simulink model "Close_Loop"  (R2019a)
settings: Solver=FixedStepDiscrete  StartTime=0.0  StopTime=100  RelTol=1e-3
libraries: simulink x5, slctrlblks x2
settings Model: Creator=markd  LastModifiedBy=lenovo
settings DebuggingCC: UnderSpecifiedDimensionMsg=warning

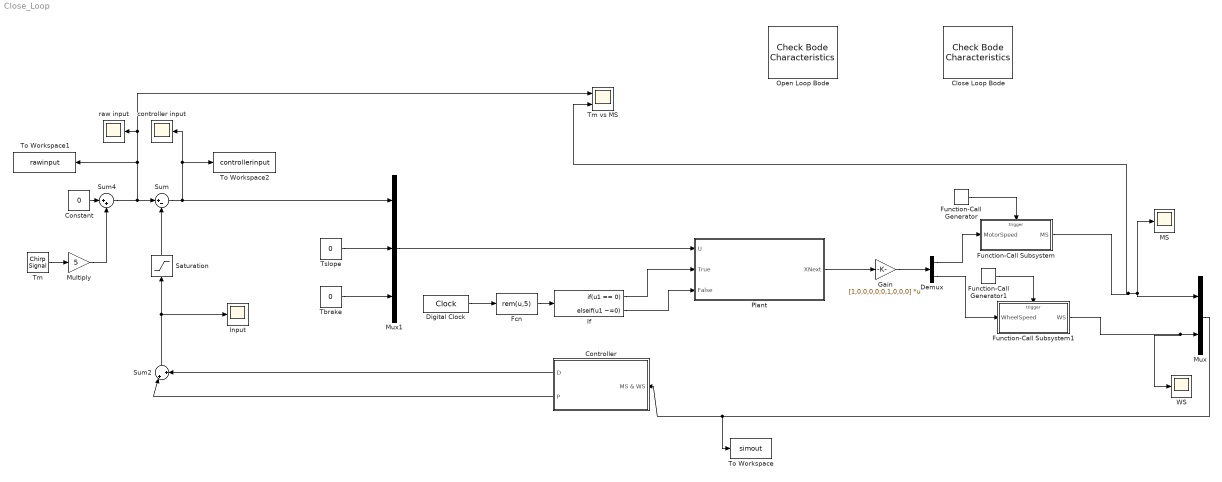
== system Close_Loop ==
  Close Loop Bode : slctrlblks/Model Verification/Check Bode  Characteristics  InstantiateOnLoad=on  SaveOperatingPoints=off  LinearizationIOs={'/Sum', 1, 'in', 'off', '';'/Demux', 1, 'out', 'off', ''}  LinearizeAt=SnapshotTimes  SnapshotTimes=[0]  TriggerType=rising  SampleTime=auto  RateConversionMethod=zoh  PreWarpFreq=10  UseExactDelayModel=off  UseFullBlockNameLabels=off  UseBusSignalLabels=off  enabled=on  stopWhenAssertionFail=off  export=off  ViewDlgPos=[1 41 1280 608]  OpenViewOnLoad=off  LaunchViewOnOpen=off  FrequencyUnits=rad/s  MagnitudeUnits=dB  PhaseUnits=deg  TimeUnits=seconds  EnableUpperBound=off  UpperBoundFrequencies=[]  UpperBoundMagnitudes=[]  EnableLowerBound=off  LowerBoundFrequencies=[]  LowerBoundMagnitudes=[]
      settings: SourceProductName=Simulink Control Design
  Constant : Constant  Value=0
  Controller : Subsystem
  Demux : Demux  Outputs=2
  Digital Clock : DigitalClock  SampleTime=0.001
  Fcn : Fcn  Expr=rem(u,5)
  Function-Call Generator : simulink/Ports & Subsystems/Function-Call Generator  sample_time=0.005  numberOfIterations=1
  Function-Call Generator1 : simulink/Ports & Subsystems/Function-Call Generator  sample_time=0.025  numberOfIterations=1
  Function-Call Subsystem : Subsystem  TreatAsAtomicUnit=on
  Function-Call Subsystem1 : Subsystem  TreatAsAtomicUnit=on
  Gain : Gain  Gain=[1,0,0,0,0;0,1,0,0,0]  Multiplication=Matrix(K*u)
  If : If  IfExpression=u1 == 0  ElseIfExpressions=u1 ~=0  ShowElse=off
  "Input " : Scope
  MS : Scope
  Multiply : Gain  Gain=5
  Mux : Mux  Inputs=2
  Mux1 : Mux  Inputs=3
  Open Loop Bode : slctrlblks/Model Verification/Check Bode  Characteristics  InstantiateOnLoad=on  SaveOperatingPoints=off  LinearizationIOs={'/Sum4', 1, 'in', 'on', '';'/Demux', 1, 'out', 'on', ''}  LinearizeAt=SnapshotTimes  SnapshotTimes=[0]  TriggerType=rising  SampleTime=auto  RateConversionMethod=zoh  PreWarpFreq=10  UseExactDelayModel=off  UseFullBlockNameLabels=off  UseBusSignalLabels=off  enabled=on  stopWhenAssertionFail=off  export=off  ViewDlgPos=[1 41 1280 608]  OpenViewOnLoad=off  LaunchViewOnOpen=off  FrequencyUnits=rad/s  MagnitudeUnits=dB  PhaseUnits=deg  TimeUnits=seconds  EnableUpperBound=off  UpperBoundFrequencies=[]  UpperBoundMagnitudes=[]  EnableLowerBound=off  LowerBoundFrequencies=[]  LowerBoundMagnitudes=[]
      settings: SourceProductName=Simulink Control Design
  Plant : Subsystem
  Saturation : Saturate  UpperLimit=50  LowerLimit=-50
  Sum : Sum  Inputs=|+-
  Sum2 : Sum  Inputs=|+|+
  Sum4 : Sum  Inputs=|++
  Tbrake : Constant  Value=0
  Tm : simulink/Sources/Chirp Signal  f1=0.1  T=100  f2=30
  Tm vs MS : Scope  NumInputPorts=2
  To Workspace : ToWorkspace  VariableName=simout  SaveFormat=Timeseries  SampleTime=-1
  To Workspace1 : ToWorkspace  VariableName=rawinput  SaveFormat=Timeseries  SampleTime=-1
  To Workspace2 : ToWorkspace  VariableName=controllerinput  SaveFormat=Timeseries  SampleTime=-1
  "Tslope " : Constant  Value=0
  WS : Scope
  controller input : Scope
  raw input : Scope
  wires:
  Tbrake/1 -> Mux1/3
  Fcn/1 -> If/1
  Digital Clock/1 -> Fcn/1
  Gain/1 -> Demux/1
  Mux1/1 -> Plant/1(U)
  If/1 -> Plant/2(True)
  If/2 -> Plant/3(False)
  Plant/1("XNext ") -> Gain/1
  Sum4/1 -> raw input/1, Tm vs MS/1, To Workspace1/1, Sum/1
  Constant/1 -> Sum4/1
  Tm/1 -> Multiply/1
  Sum/1 -> Mux1/1, controller input/1, To Workspace2/1
  "Tslope "/1 -> Mux1/2
  Multiply/1 -> Sum4/2
  Sum2/1 -> "Input "/1, Saturation/1
  Controller/1(D) -> Sum2/2
  Controller/2(P) -> Sum2/1
  Function-Call Generator/1 -> Function-Call Subsystem/Trigger
  Demux/1 -> Function-Call Subsystem/1(MotorSpeed)
  Demux/2 -> Function-Call Subsystem1/1(WheelSpeed)
  Function-Call Generator1/1 -> Function-Call Subsystem1/Trigger
  Function-Call Subsystem1/1(WS) -> WS/1, Mux/2
  Function-Call Subsystem/1(MS) -> Mux/1, MS/1, Tm vs MS/2
  Mux/1 -> To Workspace/1, Controller/1(MS & WS)
  Saturation/1 -> Sum/2

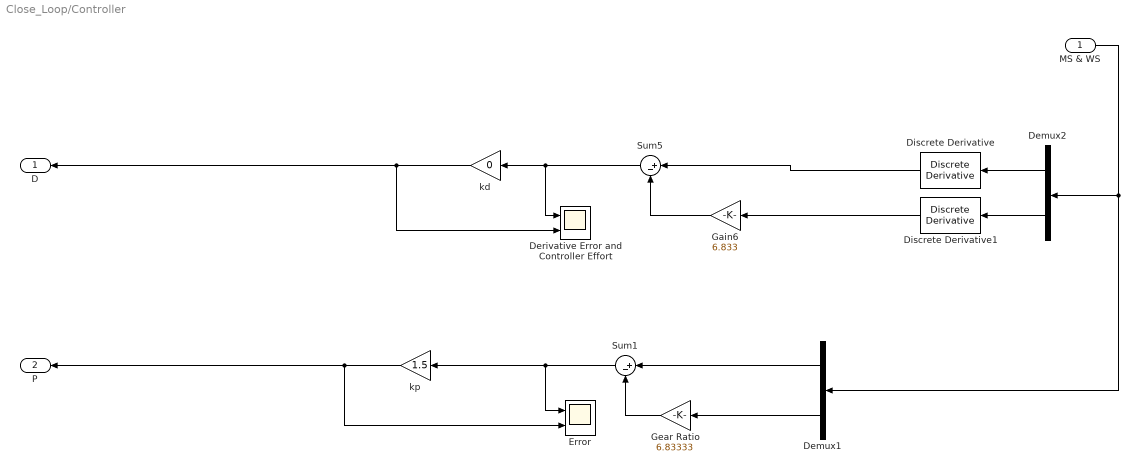
== system Close_Loop/Controller ==
  MS & WS : Inport
  Demux1 : Demux  Outputs=2
  Demux2 : Demux  Outputs=2
  Derivative Error and Controller Effort : Scope  NumInputPorts=2
  Discrete Derivative : simulink/Discrete/Discrete Derivative  gainval=1  ICPrevScaledInput=0.01*6.833  OutMin=[]  OutMax=[]  OutDataType=fixdt(1, 16)  OutScaling=2^-10  DoSatur=off
  Discrete Derivative1 : simulink/Discrete/Discrete Derivative  gainval=1  ICPrevScaledInput=0.01  OutMin=[]  OutMax=[]  OutDataType=fixdt(1, 16)  OutScaling=2^-10  DoSatur=off
  "Error " : Scope  NumInputPorts=2
  Gain6 : Gain  Gain=6.833
  Gear Ratio : Gain  Gain=6.83333
  Sum1 : Sum  Inputs=|+-
  Sum5 : Sum  Inputs=|+-
  kd : Gain  Gain=0
  kp : Gain  Gain=1.5
  D : Outport
  P : Outport  Port=2
  wires:
  MS & WS/1 -> Demux2/1, Demux1/1
  Discrete Derivative/1 -> Sum5/1
  kd/1 -> D/1, Derivative Error and Controller Effort/2
  Sum1/1 -> kp/1, "Error "/1
  Sum5/1 -> kd/1, Derivative Error and Controller Effort/1
  Demux2/1 -> Discrete Derivative/1
  Gain6/1 -> Sum5/2
  Demux2/2 -> Discrete Derivative1/1
  Gear Ratio/1 -> Sum1/2
  Discrete Derivative1/1 -> Gain6/1
  Demux1/2 -> Gear Ratio/1
  Demux1/1 -> Sum1/1
  kp/1 -> "Error "/2, P/1

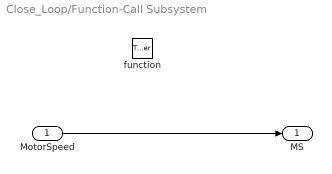
== system Close_Loop/Function-Call Subsystem ==
  MotorSpeed : Inport
  function : TriggerPort  TriggerType=function-call  VariantControl=Variant
  MS : Outport
  wires:
  MotorSpeed/1 -> MS/1

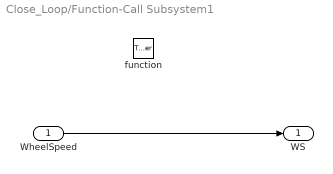
== system Close_Loop/Function-Call Subsystem1 ==
  WheelSpeed : Inport
  function : TriggerPort  TriggerType=function-call  VariantControl=Variant
  WS : Outport
  wires:
  WheelSpeed/1 -> WS/1

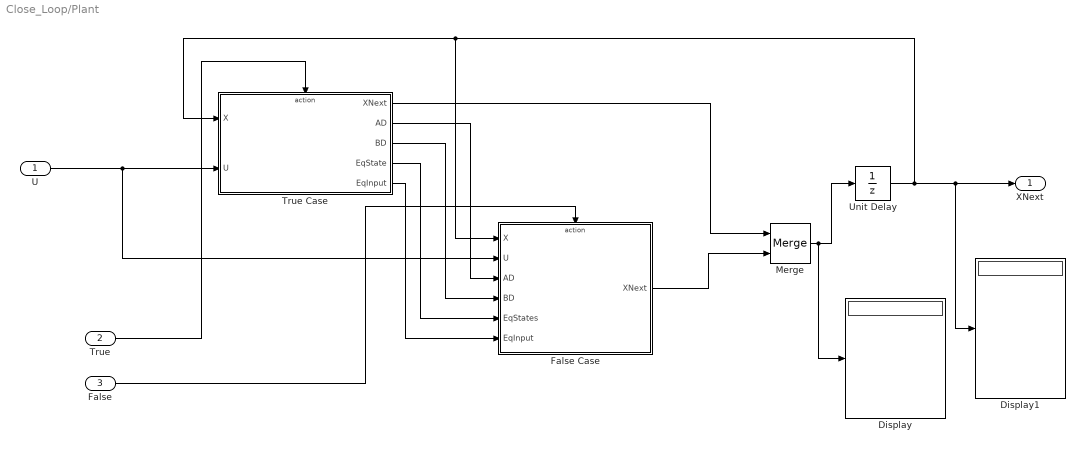
== system Close_Loop/Plant ==
  U : Inport
  True : Inport  Port=2
  False : Inport  Port=3
  Display : Display
  Display1 : Display
  False Case : Subsystem  TreatAsAtomicUnit=on
  Merge : Merge
  True Case : Subsystem  TreatAsAtomicUnit=on
  Unit Delay : UnitDelay  InitialCondition=[0.01*6.833;0.01;0.01;0;0]  SampleTime=0.001  HasFrameUpgradeWarning=on
  "XNext " : Outport
  wires:
  True Case/1(XNext) -> Merge/1
  True Case/2(AD) -> False Case/3(AD)
  Merge/1 -> Display/1, Unit Delay/1
  False Case/1(XNext) -> Merge/2
  Unit Delay/1 -> Display1/1, "XNext "/1, False Case/1(X), True Case/1(X)
  True Case/4(EqState) -> False Case/5(EqStates)
  U/1 -> True Case/2(U), False Case/2(U)
  True Case/5(EqInput) -> False Case/6(EqInput)
  True Case/3(BD) -> False Case/4(BD)
  False/1 -> False Case/Action
  True/1 -> True Case/Action

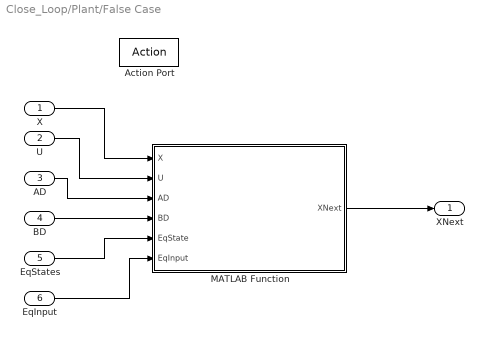
== system Close_Loop/Plant/False Case ==
  X : Inport
  U : Inport  Port=2
  AD : Inport  Port=3
  BD : Inport  Port=4
  EqStates : Inport  Port=5
  EqInput : Inport  Port=6
  Action Port : ActionPort  ActionPortLabel=elseif(u1 ~=0)
  MATLAB Function : MATLAB Function  TreatAsAtomicUnit=on
  XNext : Outport
  wires:
  MATLAB Function/1(XNext) -> XNext/1
  X/1 -> MATLAB Function/1(X)
  U/1 -> MATLAB Function/2(U)
  AD/1 -> MATLAB Function/3(AD)
  BD/1 -> MATLAB Function/4(BD)
  EqStates/1 -> MATLAB Function/5(EqState)
  EqInput/1 -> MATLAB Function/6(EqInput)

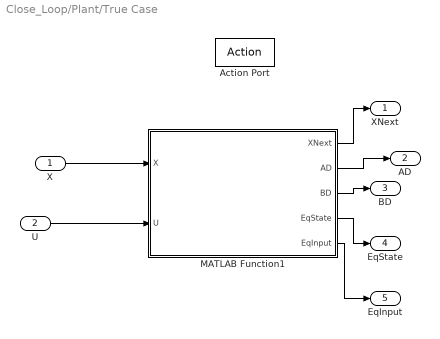
== system Close_Loop/Plant/True Case ==
  X : Inport
  U : Inport  Port=2
  Action Port : ActionPort  ActionPortLabel=if(u1 == 0)
  MATLAB Function1 : MATLAB Function  TreatAsAtomicUnit=on
  XNext : Outport
  AD : Outport  Port=2
  BD : Outport  Port=3
  EqState : Outport  Port=4
  EqInput : Outport  Port=5
  wires:
  X/1 -> MATLAB Function1/1(X)
  U/1 -> MATLAB Function1/2(U)
  MATLAB Function1/1(XNext) -> XNext/1
  MATLAB Function1/2(AD) -> AD/1
  MATLAB Function1/3(BD) -> BD/1
  MATLAB Function1/4(EqState) -> EqState/1
  MATLAB Function1/5(EqInput) -> EqInput/1

== matlab function Close_Loop/Plant/False Case/MATLAB Function ==
  data: X input; XNext output; U input; AD input; BD input; EqState input; EqInput input
function XNext = StateSpace(X,U,AD,BD,EqState,EqInput)

XNext = AD*(X-EqState)+BD*(U-EqInput)+EqState;
end

== matlab function Close_Loop/Plant/True Case/MATLAB Function1 ==
  data: X input; XNext output; U input; AD output; BD output; EqState output; EqInput output
function [XNext,AD,BD,EqState,EqInput] = StateSpace(X,U)
% Initilized the size of the matrices
% Get linearized matrices and eq points
coder.extrinsic('LinearForSim')
% Get Discretized Matrices
coder.extrinsic('StateSpace')

AD = zeros(5,5);
BD = zeros(5,3);
EqState = zeros(5,1);
EqInput = zeros(3,1);

VehicleSpeed = X(3);
Tslope = U(2);
Tbrake = U(3);

[LinearMatrix, EqPoints] = LinearForSim(VehicleSpeed,Tbrake,Tslope);
EqState = EqPoints(1:5);
EqInput = EqPoints(6:8);

[AD,BD] = StateSpace(LinearMatrix);

XNext = AD*(X-EqState)+BD*(U-EqInput)+ EqState;
  
end
